simulink model "tdm"  (R2018a)
settings: Solver=VariableStepAuto  StartTime=0.0  StopTime=8  RelTol=1e-3
libraries: simulink_extras x1
settings Model: Creator=ete  LastModifiedBy=hp
settings DataIOCC: ReturnWorkspaceOutputs=on
settings OptimizationCC: LifeSpan=inf
settings DebuggingCC: SFExecutionAtInitializationDiag=none
settings SFSimCC: SimUseLocalCustomCode=on
settings RTWCC: RTWUseLocalCustomCode=on
settings CodeAppCC: StateflowObjectComments=on
settings ConfigComp: CovHtmlReporting=on

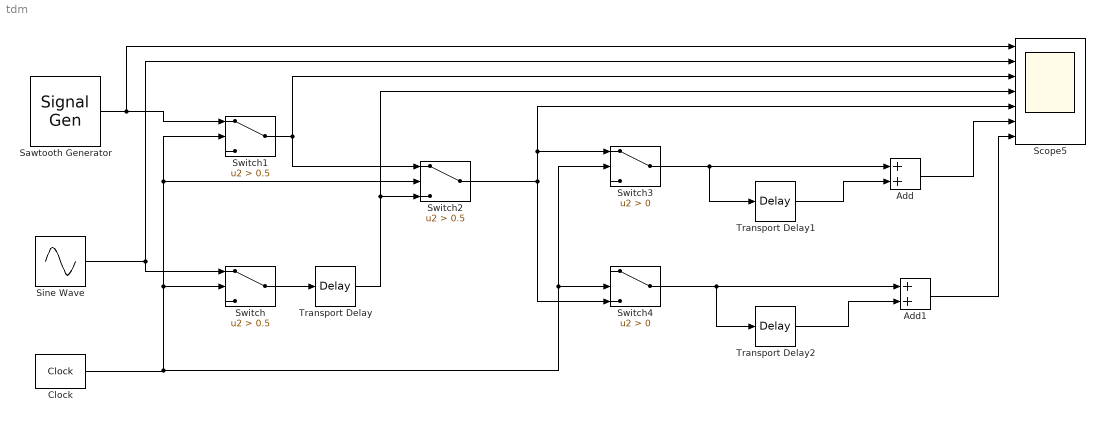
== system tdm ==
  Add : Sum
  Add1 : Sum
  Clock : simulink_extras/Flip Flops/Clock  period=2
  Sawtooth Generator : SignalGenerator  WaveForm=sawtooth  Amplitude=4  Frequency=4
  Scope5 : Scope  NumInputPorts=7
  Sine Wave : Sin  Amplitude=2  Frequency=2*pi*1  SampleTime=0.01
  Switch : Switch  Criteria=u2 > Threshold  Threshold=0.5
  Switch1 : Switch  Criteria=u2 > Threshold  Threshold=0.5
  Switch2 : Switch  Criteria=u2 > Threshold  Threshold=0.5
  Switch3 : Switch  Criteria=u2 > Threshold
  Switch4 : Switch  Criteria=u2 > Threshold
  Transport Delay : TransportDelay
  Transport Delay1 : TransportDelay
  Transport Delay2 : TransportDelay
  wires:
  Clock/1 -> Switch4/2, Switch3/2, Switch1/2, Switch2/2, Switch/2
  Sine Wave/1 -> Switch/1, Scope5/2
  Switch/1 -> Transport Delay/1
  Switch1/1 -> Scope5/3, Switch2/1
  Sawtooth Generator/1 -> Scope5/1, Switch1/1
  Switch2/1 -> Scope5/5, Switch3/1, Switch4/3
  Transport Delay/1 -> Scope5/4, Switch2/3
  Switch3/1 -> Transport Delay1/1, Add/1
  Switch4/1 -> Transport Delay2/1, Add1/1
  Transport Delay2/1 -> Add1/2
  Transport Delay1/1 -> Add/2
  Add/1 -> Scope5/6
  Add1/1 -> Scope5/7
